simulink model "sample04_speed_pd_I2C0"  (R2025b)
settings: Solver=ode1  StartTime=0.0  StopTime=inf  FixedStep=0.005  RelTol=1e-3  EnableMultiTasking=on
libraries: roller485lib x3
settings Model: ExtModeTrigDuration=2  Creator=kawata  LastModifiedBy=kawata
settings SolverCC: AutoInsertRateTranBlk=on
settings DataIOCC: ReturnWorkspaceOutputs=off
settings OptimizationCC: EnhancedBackFolding=on  PassReuseOutputArgsThreshold=0.0  MaxStackSize=64  OptimizeBlockOrder=speed  DifferentSizesBufferReuse=on  OptimizationCustomize=off
settings DebuggingCC: ParameterTunabilityLossMsg=error
settings HardwareCC: ProdBitPerPointer=32.0  ProdBitPerSizeT=32.0  ProdBitPerPtrDiffT=32.0  ProdLargestAtomicInteger=Long  ProdLargestAtomicFloat=Double  ProdWordSize=32.0  ProdHWDeviceType=ARM Compatible->ARM Cortex  UseEmbeddedCoderFeatures=off  UseSimulinkCoderFeatures=off
settings SFSimCC: MATLABDynamicMemAlloc=off
settings RTWCC: SystemTargetFile=ert.tlc  HardwareBoard=Raspberry Pi Pico (Arduino Compatible)  TemplateMakefile=ert_default_tmf  Toolchain=Arduino ARM RP2040  BuildConfiguration=Faster Runs  Description=Embedded Coder
settings CodeAppCC: ForceParamTrailComments=on  OperatorAnnotations=on
settings ERTTargetCC: ExtModeTransport=3.0  ExtModeStaticAlloc=on  ExtModeAutomaticAllocSize=off  ExtModeStaticAllocSize=65536.0  ExtModeMexFile=ext_xcp  ExtModeIntrfLevel=Level2 - Open  InlinedParameterPlacement=Hierarchical  DynamicArrayContainerType=coder::array  ERTCustomFileBanners=off  SupportContinuousTime=on  SupportNonInlinedSFcns=on  RemoveResetFunc=off  SupportVariableSizeSignals=on  ModelStepFunctionPrototypeControlCompliant=off

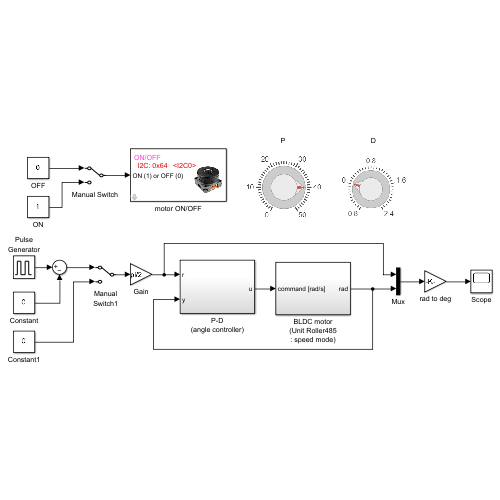
[thumbnail: Simulink's stored preview of the top-level diagram]
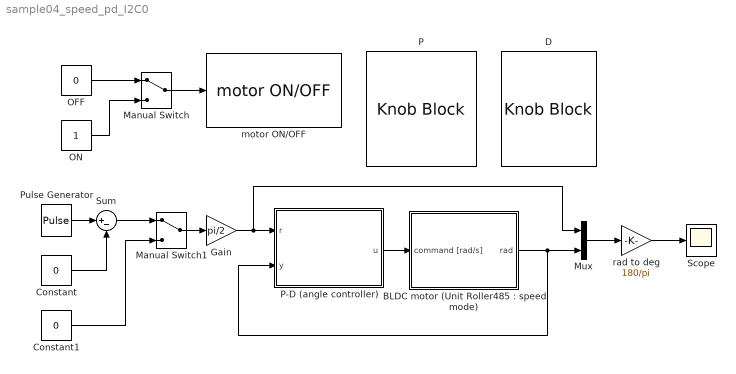
== system sample04_speed_pd_I2C0 ==
  "BLDC motor (Unit Roller485 : speed mode)" : Subsystem
  Constant : Constant  Value=0
  Constant1 : Constant  Value=0
  D : KnobBlock  LabelPosition=Hide  ScaleMin=-0.8  ScaleMax=2.4  TickInterval=0.8
  Gain : Gain  Gain=pi/2
  Manual Switch1 : ManualSwitch
  Manual Switch : ManualSwitch
  Mux : Mux  Inputs=2
  OFF : Constant  Value=0
  ON : Constant
  P : KnobBlock  LabelPosition=Hide  ScaleMax=50  TickInterval=10
  P-D (angle controller) : Subsystem
  Pulse Generator : DiscretePulseGenerator  PulseType=Time based  Period=4  PulseWidth=50  PhaseDelay=1
  Scope : Scope
      settings: TimeSpan=4  ActiveDisplayYMinimum=-45  ActiveDisplayYMaximum=135
  Sum : Sum  Inputs=|+-
  motor ON/OFF : roller485lib/motor ON//OFF  I2CAddress=0x64  I2CModule=0
      settings: SourceProductName=Roller485 Library
  rad to deg : Gain  Gain=180/pi
  wires:
  Manual Switch/1 -> motor ON/OFF/1
  OFF/1 -> Manual Switch/1
  ON/1 -> Manual Switch/2
  Constant/1 -> Sum/2
  Pulse Generator/1 -> Sum/1
  Mux/1 -> rad to deg/1
  P-D (angle controller)/1(u) -> "BLDC motor (Unit Roller485 : speed mode)"/1(command [rad/s])
  Gain/1 -> P-D (angle controller)/1(r), Mux/1
  "BLDC motor (Unit Roller485 : speed mode)"/1(rad) -> P-D (angle controller)/2(y), Mux/2
  rad to deg/1 -> Scope/1
  Manual Switch1/1 -> Gain/1
  Sum/1 -> Manual Switch1/1
  Constant1/1 -> Manual Switch1/2

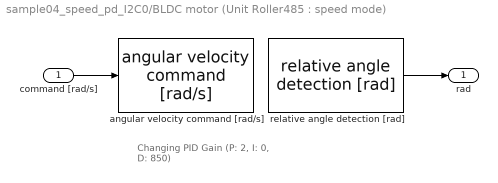
== system sample04_speed_pd_I2C0/BLDC motor (Unit Roller485 : speed mode) ==
  note: Changing PID Gain
      | (P: 2, I: 0, D: 850)
  command [rad/s] : Inport
  angular velocity command [rad/s] : roller485lib/I2C Write/angular velocity command [rad//s]  I2CAddress=0x64  I2CModule=0  speed_P=2  speed_I=0  speed_D=850  set_time1=0  set_time2=0
      settings: SourceProductName=Roller485 Library
  relative angle detection [rad] : roller485lib/I2C Read/relative angle detection [rad]  I2CAddress=0x64  I2CModule=0  sample_time=-1  set_time=0
      settings: SourceProductName=Roller485 Library
  rad : Outport
  wires:
  command [rad/s]/1 -> angular velocity command [rad/s]/1
  relative angle detection [rad]/1 -> rad/1

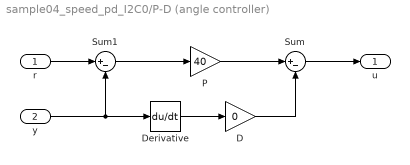
== system sample04_speed_pd_I2C0/P-D (angle controller) ==
  r : Inport
  y : Inport  Port=2
  D : Gain  Gain=0
  Derivative : Derivative
  P : Gain  Gain=40
  Sum : Sum  Inputs=|+-
  Sum1 : Sum  Inputs=|+-
  u : Outport
  wires:
  Sum/1 -> u/1
  P/1 -> Sum/1
  Derivative/1 -> D/1
  r/1 -> Sum1/1
  Sum1/1 -> P/1
  y/1 -> Sum1/2, Derivative/1
  D/1 -> Sum/2
